simulink model "sl_drivepoint"  (R2015a)
settings: Solver=ode45  StartTime=0.0  StopTime=15.0  RelTol=1e-3
undefined symbols (not defined in the file): xg
libraries: roblocks x2, simulink x1
settings Model: Creator=pic  LastModifiedBy=corkep
settings DataIOCC: LimitDataPoints=off  ReturnWorkspaceOutputs=on  TimeSaveName=t  OutputSaveName=y
settings OptimizationCC: ExpressionDepthLimit=2147483647
settings DebuggingCC: UnderspecifiedInitializationDetection=Classic  MergeDetectMultiDrivingBlocksExec=none  StateNameClashWarn=warning
settings GRTTargetCC: CombineOutputUpdateFcns=off  GRTInterface=on

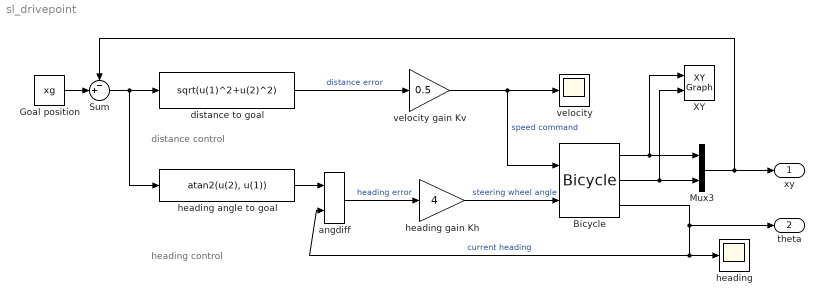
== system sl_drivepoint ==
  note: distance control
  note: heading control
  Bicycle : roblocks/Vehicles/Bicycle  vlim=1  accel=1  alim=1  steer_rate=Inf  L=1  x0=x0
  Goal position : Constant  Value=xg
  Mux3 : Mux  Inputs=2
  Sum : Sum  Inputs=-+|
  XY : simulink/Sinks/XY Graph  xmin=0  xmax=10  ymin=0  ymax=10  st=-1
  angdiff : roblocks/Toolbox/angdiff
  distance to goal : Fcn  Expr=sqrt(u(1)^2+u(2)^2)
  heading : Scope
      settings: TimeRange=auto  LimitDataPoints=on  MaxDataPoints=5000  SaveToWorkspace=off  SaveName=ScopeData  YMin=-10  YMax=10  SampleTime=-1
  heading angle to goal : Fcn  Expr=atan2(u(2), u(1))
  heading gain Kh : Gain  Gain=4
  velocity : Scope
      settings: TimeRange=auto  LimitDataPoints=on  MaxDataPoints=5000  SaveToWorkspace=off  YMin=-0.43387  YMax=3.97658  SampleTime=-1
  velocity gain Kv : Gain  Gain=0.5
  xy : Outport
  "theta " : Outport  Port=2
  wires:
  Bicycle/1 -> Mux3/1, XY/1
  Bicycle/2 -> Mux3/2, XY/2
  Mux3/1 -> Sum/1, xy/1
  Sum/1 -> distance to goal/1, heading angle to goal/1
  distance to goal/1 -> velocity gain Kv/1  "distance error"
  heading angle to goal/1 -> angdiff/1
  Bicycle/3 -> heading/1, angdiff/2, "theta "/1  "current heading"
  angdiff/1 -> heading gain Kh/1  "heading error"
  velocity gain Kv/1 -> Bicycle/1, velocity/1  "speed command"
  Goal position/1 -> Sum/2
  heading gain Kh/1 -> Bicycle/2  "steering wheel angle"
